simulink model "Integratore2"  (R2017a)
settings: Solver=VariableStepAuto  StartTime=0.0  StopTime=10.0  RelTol=1e-3
settings Model: Creator=Michele  LastModifiedBy=Michele

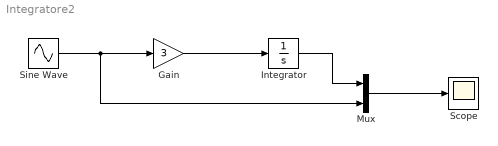
== system Integratore2 ==
  Gain : Gain  Gain=3
  Integrator : Integrator
  Mux : Mux  Inputs=2
  Scope : Scope
  Sine Wave : Sin  Frequency=2  SampleTime=0
  wires:
  Gain/1 -> Integrator/1
  Sine Wave/1 -> Mux/2, Gain/1
  Integrator/1 -> Mux/1
  Mux/1 -> Scope/1
